simulink model "misc_blocks_PQ_measurement"  (R2025a)
settings: Solver=VariableStepAuto  StartTime=0.0  StopTime=10.0  RelTol=1e-3
settings Model: Creator=atomas  LastModifiedBy=atomas

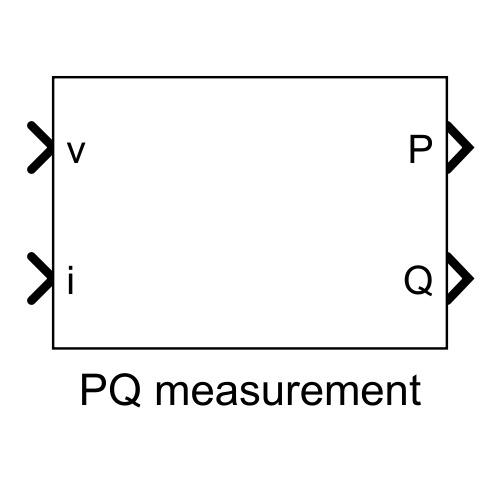
[thumbnail: Simulink's stored preview of the top-level diagram]
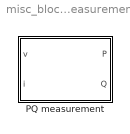
== system misc_blocks_PQ_measurement ==
  PQ measurement : Subsystem

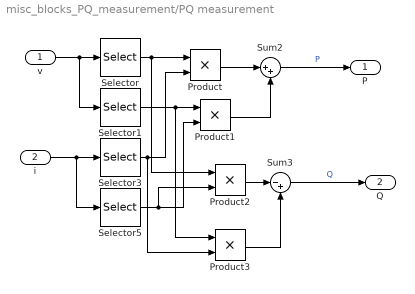
== system misc_blocks_PQ_measurement/PQ measurement ==
  v : Inport
  i : Inport  Port=2
  Product{,1..3} (4 alike) : Product
  Selector : Selector  NumberOfDimensions=2  InputPortWidth=3  IndexOptions=Index vector (dialog),Select all  Indices=1,1  OutputSizes=1,1
  Selector1 : Selector  NumberOfDimensions=2  InputPortWidth=3  IndexOptions=Index vector (dialog),Select all  Indices=2,1  OutputSizes=1,1
  Selector3 : Selector  NumberOfDimensions=2  InputPortWidth=3  IndexOptions=Index vector (dialog),Select all  Indices=1,1  OutputSizes=1,1
  Selector5 : Selector  NumberOfDimensions=2  InputPortWidth=3  IndexOptions=Index vector (dialog),Select all  Indices=2,1  OutputSizes=1,1
  Sum2 : Sum  Inputs=|++
  Sum3 : Sum  Inputs=|-+
  P : Outport
  Q : Outport  Port=2
  wires:
  Selector/1 -> Product2/1, Product/1
  i/1 -> Selector5/1, Selector3/1
  Product2/1 -> Sum3/1
  Product1/1 -> Sum2/2
  v/1 -> Selector1/1, Selector/1
  Selector3/1 -> Product3/2, Product/2
  Selector1/1 -> Product3/1, Product1/1
  Selector5/1 -> Product2/2, Product1/2
  Sum3/1 -> Q/1  "Q"
  Product/1 -> Sum2/1
  Product3/1 -> Sum3/2
  Sum2/1 -> P/1  "P"
